simulink model "WheelSpeedInputs"  (R2024b)
settings: configuration reference "STM32H7_Config" (kept outside this file)
undefined symbols (not defined in the file): rGearboxRatio, rTyreRadius
settings Model: DataDictionary=Master_Dictionary.sldd  EnableAccessToBaseWorkspace=off  Creator=torni  LastModifiedBy=Will
settings ConfigSetRef: SourceName=STM32H7_Config

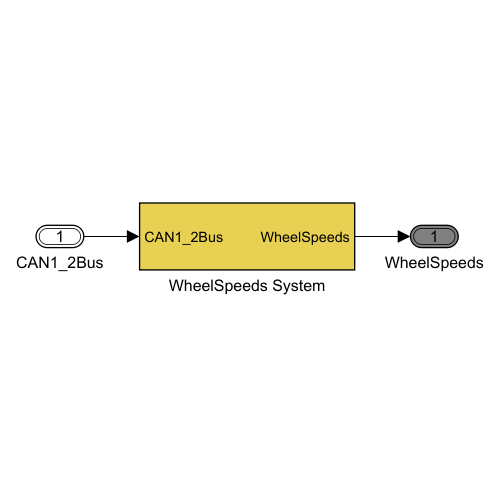
[thumbnail: Simulink's stored preview of the top-level diagram]
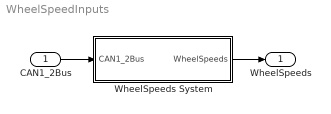
== system WheelSpeedInputs ==
  CAN1_2Bus : Inport  OutDataTypeStr=Bus: CAN1_2Bus
  WheelSpeeds System : Subsystem
  WheelSpeeds : Outport  OutDataTypeStr=Bus: WheelSpeeds  VectorParamsAs1DForOutWhenUnconnected=off
  wires:
  CAN1_2Bus/1 -> WheelSpeeds System/1(CAN1_2Bus)
  WheelSpeeds System/1(WheelSpeeds) -> WheelSpeeds/1

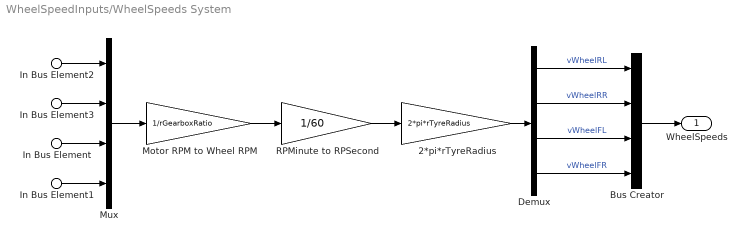
== system WheelSpeedInputs/WheelSpeeds System ==
  In Bus Element : Inport  PortName=CAN1_2Bus  Element=InverterFL.nMotorFL
  In Bus Element1 : Inport  PortName=CAN1_2Bus  Element=InverterFR.nMotorFR
  In Bus Element2 : Inport  PortName=CAN1_2Bus  Element=InverterRL.nMotorRL
  In Bus Element3 : Inport  PortName=CAN1_2Bus  Element=InverterRR.nMotorRR
  2*pi*rTyreRadius : Gain  Gain=2*pi*rTyreRadius
  Bus Creator : BusCreator  Inputs=4  OutDataTypeStr=Bus: WheelSpeeds
  Demux : Demux
  Motor RPM to Wheel RPM : Gain  Gain=1/rGearboxRatio
  Mux : Mux
  RPMinute to RPSecond : Gain  Gain=1/60
  WheelSpeeds : Outport  OutDataTypeStr=Bus: WheelSpeeds  VectorParamsAs1DForOutWhenUnconnected=off
  wires:
  Demux/1 -> Bus Creator/1  "vWheelRL"
  Demux/2 -> Bus Creator/2  "vWheelRR"
  Demux/4 -> Bus Creator/4  "vWheelFR"
  Demux/3 -> Bus Creator/3  "vWheelFL"
  In Bus Element2/1 -> Mux/1
  In Bus Element3/1 -> Mux/2
  In Bus Element/1 -> Mux/3
  In Bus Element1/1 -> Mux/4
  RPMinute to RPSecond/1 -> 2*pi*rTyreRadius/1
  Mux/1 -> Motor RPM to Wheel RPM/1
  Motor RPM to Wheel RPM/1 -> RPMinute to RPSecond/1
  2*pi*rTyreRadius/1 -> Demux/1
  Bus Creator/1 -> WheelSpeeds/1
